simulink model "Gravity_Drained_Tanks_Test_WCPSv4"  (R2018a)
settings: Solver=ode45  StartTime=0.0  StopTime=10000  RelTol=1e-3  EnableMultiTasking=on
PreLoadFcn:
  | Initialize
StopFcn:
  | Plot_and_save
values from neighbouring files (symbols this model uses):
  delta_t = 10    [Initialize.m]
  delta_t_moter = 10    [Initialize.m]
undefined symbols (not defined in the file or in its folder): P
libraries: simulink x5
settings Model: Creator=tsladeche  LastModifiedBy=root
settings DataIOCC: LimitDataPoints=on  SaveFormat=Array  SignalLoggingSaveFormat=ModelDataLogs
settings OptimizationCC: ExpressionDepthLimit=2147483647  LifeSpan=inf
settings DebuggingCC: UnderspecifiedInitializationDetection=Classic  MergeDetectMultiDrivingBlocksExec=none  SolverPrmCheckMsg=warning  FcnCallInpInsideContextMsg=warning  StateNameClashWarn=warning  SFUnexpectedBacktrackingDiag=warning  SFNoUnconditionalDefaultTransitionDiag=warning  SFExecutionAtInitializationDiag=none
settings HardwareCC: ProdBitPerPointer=32  ProdBitPerSizeT=32  ProdBitPerPtrDiffT=32  ProdLargestAtomicFloat=None  ProdIntDivRoundTo=Undefined  ProdEndianess=Unspecified  ProdWordSize=32  ProdHWDeviceType=32-bit Generic
settings ModelReferenceCC: PropagateSignalLabelsOutOfModel=off
settings CodeAppCC: StateflowObjectComments=on
settings GRTTargetCC: TargetLangStandard=C89/C90 (ANSI)  GeneratePreprocessorConditionals=Disable all  CombineOutputUpdateFcns=off  GRTInterface=on
settings ConfigComp: CovMetricSettings=dw  CovHtmlReporting=on  CovSaveCumulativeToWorkspaceVar=on  CovSaveSingleToWorkspaceVar=on  CovExternalEMLEnable=off  CovSFcnEnable=off

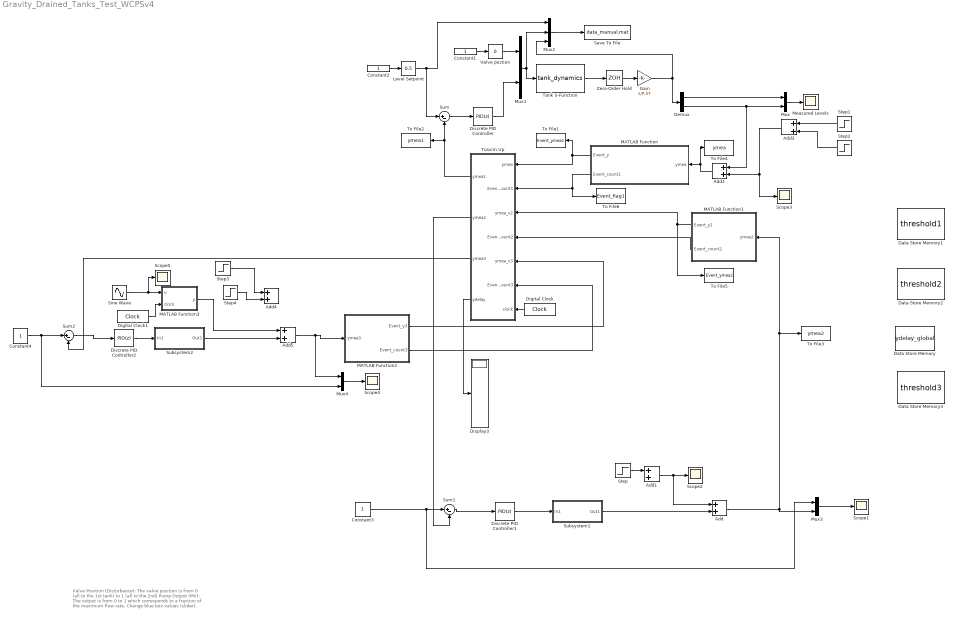
== system Gravity_Drained_Tanks_Test_WCPSv4 ==
  note: Valve Position (Disturbance): The valve position is from
      | 0 (all to the 1st tank) to 1 (all to the 2nd)
      |
      | Pump Output (MV): The output is from 0 to 1 which
      | corresponds to a fraction of the maximum flow rate.
      |
      | Change blue box values (slider).
  Add{,1..5} (6 alike) : Sum
  Constant{1..4} (4 alike) : Constant
  Data Store Memory : DataStoreMemory  DataStoreName=ydelay_global  ReadBeforeWriteMsg=warning  WriteAfterWriteMsg=warning  WriteAfterReadMsg=warning  InitialValue=[1; 1; 1; 1; 1; 1; 1; 1; 1; 1; 1; 1; 1; 1; 1]  ShowAdditionalParam=off  OutDataTypeStr=uint32
  Data Store Memory1 : DataStoreMemory  DataStoreName=threshold1  ReadBeforeWriteMsg=warning  WriteAfterWriteMsg=warning  WriteAfterReadMsg=warning  InitialValue=th1_initial  ShowAdditionalParam=off  OutDataTypeStr=double
  Data Store Memory2 : DataStoreMemory  DataStoreName=threshold2  ReadBeforeWriteMsg=warning  WriteAfterWriteMsg=warning  WriteAfterReadMsg=warning  InitialValue=th2_initial  ShowAdditionalParam=off  OutDataTypeStr=double
  Data Store Memory3 : DataStoreMemory  DataStoreName=threshold3  ReadBeforeWriteMsg=warning  WriteAfterWriteMsg=warning  WriteAfterReadMsg=warning  InitialValue=th2_initial  ShowAdditionalParam=off  OutDataTypeStr=double
  Demux : Demux  Outputs=2
  Digital Clock : DigitalClock  SampleTime=delta_t
  Digital Clock1 : DigitalClock  SampleTime=delta_t
  Discrete PID Controller : simulink/Continuous/PID Controller  Controller=PID  TimeDomain=Discrete-time  SampleTime=delta_t  IntegratorMethod=Forward Euler  FilterMethod=Forward Euler  Form=Parallel  UseFilter=on  ControllerParametersSource=internal  P=1/1.624181124  I=(1/1.624181124)/140.7309944  D=0  N=100  InitialConditionSource=internal  InitialConditionForIntegrator=0  InitialConditionForFilter=0  ExternalReset=none  LimitOutput=on  UpperSaturationLimit=1  LowerSaturationLimit=0  LinearizeAsGain=on  AntiWindupMode=clamping  Kb=1  TrackingMode=off  Kt=1  PParamMin=[]  PParamMax=[]  IParamMin=[]  IParamMax=[]  DParamMin=[]  DParamMax=[]  NParamMin=[]  NParamMax=[]  KbParamMin=[]  KbParamMax=[]  KtParamMin=[]  KtParamMax=[]  POutMin=[]  POutMax=[]  IOutMin=[]  IOutMax=[]  DOutMin=[]  DOutMax=[]  NOutMin=[]  NOutMax=[]  KbOutMin=[]  KbOutMax=[]  KtOutMin=[]  KtOutMax=[]  IntegratorOutMin=[]  IntegratorOutMax=[]  FilterOutMin=[]  FilterOutMax=[]  SumOutMin=[]  SumOutMax=[]  SumI1OutMin=[]  SumI1OutMax=[]  SumI2OutMin=[]  SumI2OutMax=[]  SumI3OutMin=[]  SumI3OutMax=[]  SumDOutMin=[]  SumDOutMax=[]  SaturationOutMin=[]  SaturationOutMax=[]  IntegratorContinuousStateAttributes=''  IntegratorStateMustResolveToSignalObject=off  IntegratorRTWStateStorageClass=Auto  FilterContinuousStateAttributes=''  FilterStateMustResolveToSignalObject=off  FilterRTWStateStorageClass=Auto  DifferentiatorICPrevScaledInput=0  DifferentiatorOutMin=[]  DifferentiatorOutMax=[]  FilterDiffOutCoefMin=[]  FilterDiffOutCoefMax=[]  SumDenOutMin=[]  SumDenOutMax=[]  SumNumOutMin=[]  SumNumOutMax=[]  ReciprocalOutMin=[]  ReciprocalOutMax=[]  DivideOutMin=[]  DivideOutMax=[]  TunerSelectOption=Transfer Function Based (PID Tuner App)
  Discrete PID Controller1 : simulink/Continuous/PID Controller  Controller=PID  TimeDomain=Discrete-time  SampleTime=delta_t_moter  IntegratorMethod=Forward Euler  FilterMethod=Forward Euler  Form=Parallel  UseFilter=on  ControllerParametersSource=internal  P=0.0705520945054552  I=0.014110418901091  D=0  N=100  InitialConditionSource=internal  InitialConditionForIntegrator=0  InitialConditionForFilter=0  ExternalReset=none  LimitOutput=off  UpperSaturationLimit=inf  LowerSaturationLimit=-inf  LinearizeAsGain=off  AntiWindupMode=none  Kb=1  TrackingMode=off  Kt=1  PParamMin=[]  PParamMax=[]  IParamMin=[]  IParamMax=[]  DParamMin=[]  DParamMax=[]  NParamMin=[]  NParamMax=[]  KbParamMin=[]  KbParamMax=[]  KtParamMin=[]  KtParamMax=[]  POutMin=[]  POutMax=[]  IOutMin=[]  IOutMax=[]  DOutMin=[]  DOutMax=[]  NOutMin=[]  NOutMax=[]  KbOutMin=[]  KbOutMax=[]  KtOutMin=[]  KtOutMax=[]  IntegratorOutMin=[]  IntegratorOutMax=[]  FilterOutMin=[]  FilterOutMax=[]  SumOutMin=[]  SumOutMax=[]  SumI1OutMin=[]  SumI1OutMax=[]  SumI2OutMin=[]  SumI2OutMax=[]  SumI3OutMin=[]  SumI3OutMax=[]  SumDOutMin=[]  SumDOutMax=[]  SaturationOutMin=[]  SaturationOutMax=[]  IntegratorContinuousStateAttributes=''  IntegratorStateMustResolveToSignalObject=off  IntegratorRTWStateStorageClass=Auto  FilterContinuousStateAttributes=''  FilterStateMustResolveToSignalObject=off  FilterRTWStateStorageClass=Auto  DifferentiatorICPrevScaledInput=0  DifferentiatorOutMin=[]  DifferentiatorOutMax=[]  FilterDiffOutCoefMin=[]  FilterDiffOutCoefMax=[]  SumDenOutMin=[]  SumDenOutMax=[]  SumNumOutMin=[]  SumNumOutMax=[]  ReciprocalOutMin=[]  ReciprocalOutMax=[]  DivideOutMin=[]  DivideOutMax=[]  TunerSelectOption=Transfer Function Based (PID Tuner App)
  Discrete PID Controller2 : simulink/Continuous/PID Controller  Controller=PID  TimeDomain=Discrete-time  SampleTime=delta_t_moter  IntegratorMethod=Forward Euler  FilterMethod=Forward Euler  Form=Parallel  UseFilter=on  ControllerParametersSource=internal  P=0.0705520945054552  I=0.014110418901091  D=0  N=100  InitialConditionSource=internal  InitialConditionForIntegrator=0  InitialConditionForFilter=0  ExternalReset=none  LimitOutput=off  UpperSaturationLimit=inf  LowerSaturationLimit=-inf  LinearizeAsGain=off  AntiWindupMode=none  Kb=1  TrackingMode=off  Kt=1  PParamMin=[]  PParamMax=[]  IParamMin=[]  IParamMax=[]  DParamMin=[]  DParamMax=[]  NParamMin=[]  NParamMax=[]  KbParamMin=[]  KbParamMax=[]  KtParamMin=[]  KtParamMax=[]  POutMin=[]  POutMax=[]  IOutMin=[]  IOutMax=[]  DOutMin=[]  DOutMax=[]  NOutMin=[]  NOutMax=[]  KbOutMin=[]  KbOutMax=[]  KtOutMin=[]  KtOutMax=[]  IntegratorOutMin=[]  IntegratorOutMax=[]  FilterOutMin=[]  FilterOutMax=[]  SumOutMin=[]  SumOutMax=[]  SumI1OutMin=[]  SumI1OutMax=[]  SumI2OutMin=[]  SumI2OutMax=[]  SumI3OutMin=[]  SumI3OutMax=[]  SumDOutMin=[]  SumDOutMax=[]  SaturationOutMin=[]  SaturationOutMax=[]  IntegratorContinuousStateAttributes=''  IntegratorStateMustResolveToSignalObject=off  IntegratorRTWStateStorageClass=Auto  FilterContinuousStateAttributes=''  FilterStateMustResolveToSignalObject=off  FilterRTWStateStorageClass=Auto  DifferentiatorICPrevScaledInput=0  DifferentiatorOutMin=[]  DifferentiatorOutMax=[]  FilterDiffOutCoefMin=[]  FilterDiffOutCoefMax=[]  SumDenOutMin=[]  SumDenOutMax=[]  SumNumOutMin=[]  SumNumOutMax=[]  ReciprocalOutMin=[]  ReciprocalOutMax=[]  DivideOutMin=[]  DivideOutMax=[]  TunerSelectOption=Transfer Function Based (PID Tuner App)
  Display3 : Display
  Gain : Gain  Gain=1/P.hT
  Level Setpoint : simulink/Math Operations/Slider Gain  gain=0.5  low=0  high=1
  MATLAB Function : MATLAB Function  TreatAsAtomicUnit=on
  MATLAB Function1 : MATLAB Function  TreatAsAtomicUnit=on
  MATLAB Function2 : MATLAB Function  TreatAsAtomicUnit=on
  MATLAB Function3 : MATLAB Function  TreatAsAtomicUnit=on
  Measured Levels : Scope
  Mux{,1,3..4} (4 alike) : Mux  Inputs=2
  Mux2 : Mux  Inputs=3
  Save To File : ToFile  Filename=data_manual.mat  MatrixName=tanks  SampleTime=1
  Scope{1..5} (5 alike) : Scope
  Sine Wave : Sin  Amplitude=0.2  Frequency=0.005  SampleTime=delta_t_moter
  Step : Step  Time=3000  After=0.1  SampleTime=delta_t_moter
  Step1 : Step  Time=3000  After=-0.1  SampleTime=delta_t_moter
  Step2 : Step  Time=3300  After=0.1  SampleTime=delta_t_moter
  Step3 : Step  Time=3000  After=0.1  SampleTime=delta_t_moter
  Step4 : Step  Time=3100  After=-0.2  SampleTime=delta_t_moter
  Subsystem1 : Subsystem
  Subsystem2 : Subsystem
  Sum : Sum  Inputs=|+-
  Sum1 : Sum  Inputs=|+-
  Sum2 : Sum  Inputs=|+-
  Tank S-Function : S-Function  FunctionName=tank_dynamics  Parameters=P  SFunctionDeploymentMode=off  EnableBusSupport=off
  To File1 : ToFile  Filename=Event_ymea1  MatrixName=Event_ymea1  SampleTime=delta_t
  To File2 : ToFile  Filename=ymea1  MatrixName=ymea1  SampleTime=delta_t
  To File3 : ToFile  Filename=ymea2  MatrixName=ymea2  SampleTime=delta_t_moter
  To File4 : ToFile  Filename=ymea  MatrixName=ymea  SampleTime=delta_t
  To File5 : ToFile  Filename=Event_ymea2  MatrixName=Event_ymea2  SampleTime=delta_t_moter
  To File6 : ToFile  Filename=Event_flag1  MatrixName=Event_flag1  SampleTime=delta_t
  Tossim Up : MATLAB Function  TreatAsAtomicUnit=on
  Valve postion : simulink/Math Operations/Slider Gain  gain=0  low=0  high=1
  Zero-Order Hold : ZeroOrderHold  SampleTime=delta_t
  wires:
  Gain/1 -> Demux/1, Mux2/3
  Mux2/1 -> Save To File/1
  Constant1/1 -> Valve postion/1
  Mux1/1 -> Mux2/2, Tank S-Function/1
  Valve postion/1 -> Mux1/1
  Constant2/1 -> Level Setpoint/1
  Level Setpoint/1 -> Sum/1, Mux2/1
  Mux/1 -> Measured Levels/1
  Demux/1 -> Mux/1
  Demux/2 -> Add2/1, Mux/2
  Sum/1 -> Discrete PID Controller/1
  Discrete PID Controller/1 -> Mux1/2
  Tank S-Function/1 -> Zero-Order Hold/1
  Zero-Order Hold/1 -> Gain/1
  Digital Clock/1 -> Tossim Up/7(clock)
  Tossim Up/4(ydelay) -> Display3/1
  MATLAB Function/1(Event_y) -> Tossim Up/1(ymea), To File1/1
  Tossim Up/1(ymea1) -> Sum/2, To File2/1
  MATLAB Function1/1(Event_y2) -> Tossim Up/3(ymea_v2), To File5/1
  Mux3/1 -> Scope1/1
  Constant3/1 -> Mux3/1, Sum1/1
  Sum1/1 -> Discrete PID Controller1/1
  Discrete PID Controller1/1 -> Subsystem1/1(In1)
  Tossim Up/2(ymea2) -> Sum1/2
  Subsystem1/1(Out1) -> Add/2
  Add/1 -> MATLAB Function1/1(ymea2), To File3/1, Mux3/2
  Step/1 -> Add1/1
  Add1/1 -> Add/1, Scope2/1
  Add3/1 -> Add2/2, Scope3/1
  Step1/1 -> Add3/1
  Add2/1 -> To File4/1, MATLAB Function/1(ymea)
  Step2/1 -> Add3/2
  MATLAB Function/2(Event_count1) -> To File6/1, Tossim Up/2(Event_count1)
  MATLAB Function1/2(Event_count2) -> Tossim Up/4(Event_count2)
  Sum2/1 -> Discrete PID Controller2/1
  Discrete PID Controller2/1 -> Subsystem2/1(In1)
  Constant4/1 -> Mux4/2, Sum2/1
  Mux4/1 -> Scope4/1
  MATLAB Function2/1(Event_y3) -> Tossim Up/5(ymea_v3)
  MATLAB Function2/2(Event_count3) -> Tossim Up/6(Event_count3)
  Tossim Up/3(ymea3) -> Sum2/2
  Step3/1 -> Add4/1
  Step4/1 -> Add4/2
  Subsystem2/1(Out1) -> Add5/2
  Add5/1 -> Mux4/1, MATLAB Function2/1(ymea3)
  Sine Wave/1 -> Scope5/1, MATLAB Function3/1(u)
  Digital Clock1/1 -> MATLAB Function3/2(clock)
  MATLAB Function3/1(y) -> Add5/1

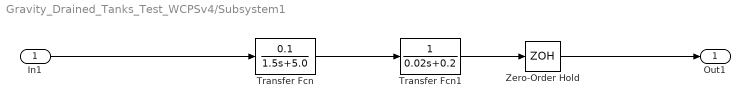
== system Gravity_Drained_Tanks_Test_WCPSv4/Subsystem1 ==
  In1 : Inport
  Transfer Fcn : TransferFcn  Numerator=[0.1]  Denominator=[1.5 5.0]
  Transfer Fcn1 : TransferFcn  Denominator=[0.02 0.2]
  Zero-Order Hold : ZeroOrderHold  SampleTime=delta_t_moter
  Out1 : Outport
  wires:
  Transfer Fcn/1 -> Transfer Fcn1/1
  In1/1 -> Transfer Fcn/1
  Transfer Fcn1/1 -> Zero-Order Hold/1
  Zero-Order Hold/1 -> Out1/1

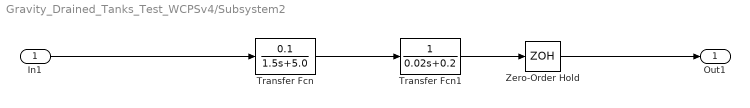
== system Gravity_Drained_Tanks_Test_WCPSv4/Subsystem2 ==
  In1 : Inport
  Transfer Fcn : TransferFcn  Numerator=[0.1]  Denominator=[1.5 5.0]
  Transfer Fcn1 : TransferFcn  Denominator=[0.02 0.2]
  Zero-Order Hold : ZeroOrderHold  SampleTime=delta_t_moter
  Out1 : Outport
  wires:
  Transfer Fcn/1 -> Transfer Fcn1/1
  In1/1 -> Transfer Fcn/1
  Transfer Fcn1/1 -> Zero-Order Hold/1
  Zero-Order Hold/1 -> Out1/1

== matlab function Gravity_Drained_Tanks_Test_WCPSv4/Tossim Up ==
  settings: updateMethod=DISCRETE
  data: ymea1 output; ymea2 output; ymea3 output; ymea input; Event_count1 input; ydelay output; ydelay_global data_store_memory; ymea_v2 input; Event_count2 input; ymea_v3 input; Event_count3 input; clock input
function [ymea1,ymea2,ymea3 ,ydelay]  = Tossim_block(ymea, Event_count1, ymea_v2,Event_count2, ymea_v3, Event_count3,clock)
% Inputs:
% ymea: measurement from structure
% Outputs:
% ymea1: measurement output
% ydelay: delay traces
persistent delay1 past_ymea past_ymea_v2 past_ymea_v3 % delay trace
persistent new_trans_ymea new_trans_ymea_v2
persistent i Task_period % count 
global ydelay_global 


% allow these matlab functions to be used in Embedded Matlab block
eml.extrinsic('python');
eml.extrinsic('num2str');
eml.extrinsic('str2num');
eml.extrinsic('delay_summary');
eml.extrinsic('disp');
eml.extrinsic('ps_aggregation');
eml.extrinsic('for');
eml.extrinsic('end');

if isempty(i)
    i = 0;
    %past_ymea = 0;
    past_ymea = ymea;
    past_ymea_v2 = ymea_v2;
    past_ymea_v3 = ymea_v3;
    new_trans_ymea = 0;
    new_trans_ymea_v2 = 0;
    Task_period = [10 10 8];        %Task_period=[10 10 4] * 10
end

%[row column] = size(Task_period_time);

ydelay = [1 0 0 0 0 0 0 0 0]';
% call python to communicate with TOSSIM

call_count = 1; %Superframelength
rssi = -69;%sensor rssi
%Total_Event_count = [Event_count1 Event_count2]

%%***
[resultz] = ps_aggregation(call_count, Event_count1, Event_count2, Event_count3);%here call TOSSIM Client ----yh
end_to_end_delivery_result_aggregated = sum(resultz)

resultz

%[delay] = delay_summary(end_to_end_delivery_result_aggregated);
[delay] = delay_summary(resultz);

delay

% for event trigger!!!
Task_period_time = Task_period * 10



ydelay = delay';

delay1 = ydelay;
x =ydelay(2);
i = i+1;

%ymea1 = ymea;

for i_yg = 1:9
    ydelay_global(i_yg, 1) = ydelay(i_yg, 1);
end
delay = ydelay';


ymea_v1_index = 1;
ymea_v2_index = 2;
ymea_v3_index = 3;

%{
if rem(clock,Task_period_time(1,2)) == 0 && ymea_v2_index == 2
    new_trans_ymea_v2 = ymea_v2;
end
if rem(clock,Task_period_time(1,1)) == 0 && ymea_v1_index == 1
    new_trans_ymea = ymea;
end
%}
%{
if delay(1,ymea_v1_index + 1)~=88
    ymea1 = past_ymea;
    %ymea1 = new_trans_ymea;
    past_ymea = ymea;
    %%%%
    ymea2 = past_ymea_v2;
    ymea3 = past_ymea_v3;
elseif delay(1,ymea_v2_index + 1)~=88
    ymea2 = past_ymea_v2;
    %ymea2 = new_trans_ymea_v2;
    past_ymea_v2 = ymea_v2;
    %%%
    ymea1 = past_ymea;
    ymea3 = past_ymea_v3;
elseif delay(1,ymea_v3_index + 1)~=88
    ymea3 = past_ymea_v3;
    past_ymea_v3 = ymea_v3;
    %%%
    ymea1 = past_ymea;
    ymea2 = past_ymea_v2;
else
    ymea1 = past_ymea;
    ymea2 = past_ymea_v2;
    ymea3 = past_ymea_v3;
end
%}
if delay(1,ymea_v1_index + 1)~=88
    ans1 = past_ymea;
    %ymea1 = new_trans_ymea;
    past_ymea = ymea;
    %%%%
    ans2 = past_ymea_v2;
    ans3 = past_ymea_v3;
elseif delay(1,ymea_v2_index + 1)~=88
    ans2 = past_ymea_v2;
    %ymea2 = new_trans_ymea_v2;
    past_ymea_v2 = ymea_v2;
    %%%
    ans1 = past_ymea;
    ans3 = past_ymea_v3;
elseif delay(1,ymea_v3_index + 1)~=88
    ans3 = past_ymea_v3;
    past_ymea_v3 = ymea_v3;
    %%%
    ans1 = past_ymea;
    ans2 = past_ymea_v2;
else
    ans1 = past_ymea;
    ans2 = past_ymea_v2;
    ans3 = past_ymea_v3;
end

ymea1 = ans1;
ymea2 = ans2;
ymea3 = ans3;

== matlab function Gravity_Drained_Tanks_Test_WCPSv4/MATLAB Function ==
  data: ymea input; Event_y output; threshold1 data_store_memory; Event_count1 output
function [Event_y, Event_count1] = event_trigger(ymea)

persistent previous_ymea tmpflag
persistent i %count
global threshold1


if isempty(i)
    i = 0;
    tmpflag = 0;
    previous_ymea = 0;
end

compare = abs(ymea - previous_ymea);
if (compare) >= threshold1
    ans = ymea;
    previous_ymea = ymea;
    tmpflag = tmpflag + 1;
else
    ans = previous_ymea;
    %tmpflag = 0;
end

i = i + 1;
Event_count1 = tmpflag;
Event_y = ans;

== matlab function Gravity_Drained_Tanks_Test_WCPSv4/MATLAB Function1 ==
  data: ymea2 input; Event_y2 output; threshold2 data_store_memory; Event_count2 output
function [Event_y2, Event_count2] = event_trigger2(ymea2)

persistent previous_ymea tmpflag
persistent i %count
global threshold2


if isempty(i)
    i = 0;
    tmpflag = 0;
    previous_ymea = 0;
end

compare = abs(ymea2 - previous_ymea);
if (compare) >= threshold2
    ans = ymea2;
    previous_ymea = ymea2;
    tmpflag = tmpflag + 1;
else
    ans = previous_ymea;
end

i = i + 1;
Event_count2 = tmpflag;
Event_y2 = ans;

== matlab function Gravity_Drained_Tanks_Test_WCPSv4/MATLAB Function2 ==
  data: ymea3 input; Event_y3 output; threshold3 data_store_memory; Event_count3 output
function [Event_y3, Event_count3] = event_trigger3(ymea3)

persistent previous_ymea tmpflag
persistent i %count
global threshold3


if isempty(i)
    i = 0;
    tmpflag = 0;
    previous_ymea = 0;
end

compare = abs(ymea3 - previous_ymea);
if (compare) >= threshold3
    ans = ymea3;
    previous_ymea = ymea3;
    tmpflag = tmpflag + 1;
else
    ans = previous_ymea;
end

i = i + 1;
Event_count3 = tmpflag;
Event_y3 = ans;

== matlab function Gravity_Drained_Tanks_Test_WCPSv4/MATLAB Function3 ==
  data: u input; y output; clock input
function y = fcn(u, clock)

if clock>3000 && clock < 3500
    y = u;
else
    y = 0;
end
